simulink subsystem "Charger"  (R2023a)
settings: Solver=VariableStepAuto  StartTime=0.0  StopTime=10.0  RelTol=1e-3
undefined symbols (not defined in the file): SRE, ts
libraries: fl_lib x2, simulink x1, nesl_utility_internal x1
settings Model: Creator=The MathWorks, Inc.  LastModifiedBy=The MathWorks, Inc.
settings SolverCC: AlgebraicLoopSolver=TrustRegion  MaxZcPerStep=1
settings OptimizationCC: ReuseModelBlockBuffer=off
settings DebuggingCC: UnconnectedInputMsg=warning  UnconnectedOutputMsg=warning  UnconnectedLineMsg=warning
settings ModelReferenceCC: EnableRefExpFcnMdlSchedulingChecks=on
settings RTWCC: DLArmComputeVersion=19.05

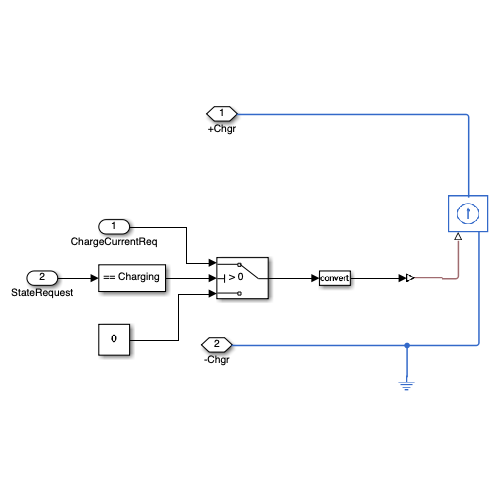
[thumbnail: Simulink's stored preview of the top-level diagram]
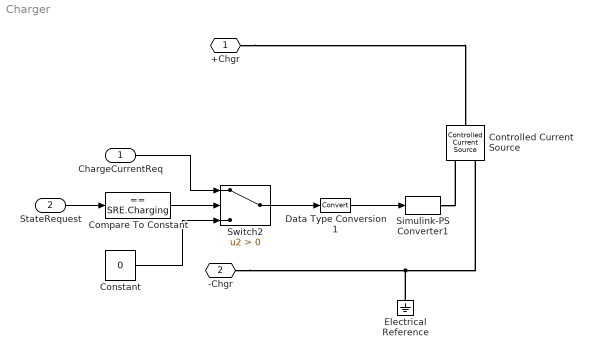
== system Charger ==
  ChargeCurrentReq : Inport
  StateRequest : Inport  Port=2
  Compare To Constant : simulink/Logic and Bit Operations/Compare To Constant  relop===  const=SRE.Charging  OutDataTypeStr=boolean
  Constant : Constant  Value=0  SampleTime=ts
  Controlled Current Source : fl_lib/Electrical/Electrical Sources/Controlled Current Source
      settings: SourceProductName=Foundation Library  LogSimulationData=on
  Data Type Conversion1 : DataTypeConversion  SaturateOnIntegerOverflow=off  RndMeth=Floor
  Electrical Reference : fl_lib/Electrical/Electrical Elements/Electrical Reference
      settings: SourceProductName=Foundation Library
  Simulink-PS Converter1 : nesl_utility_internal/Simulink-PS Converter  PhysicalDomain=network_engine_domain  SubClassName=ps_input  LeftPortType=input  RightPortType=output  PseudoPeriodic=off  Frequencies=[]  NoiseDistribution=none  NoiseParameters=[]  Unit=1  AffineConversion=off  FilteringAndDerivatives=zero  SimscapeFilterOrder=1  InputFilterTimeConstant=0.001  UdotUserProvided=1
  Switch2 : Switch  Criteria=u2 > Threshold  SaturateOnIntegerOverflow=off  InputSameDT=off
  +Chgr : PMIOPort  Side=Left
  -Chgr : PMIOPort  Port=2  Side=Left
  wires:
  Switch2/1 -> Data Type Conversion1/1
  StateRequest/1 -> Compare To Constant/1
  ChargeCurrentReq/1 -> Switch2/1
  Compare To Constant/1 -> Switch2/2
  Data Type Conversion1/1 -> Simulink-PS Converter1/1
  Constant/1 -> Switch2/3
  connections:
  Controlled Current Source/RConn2 -- -Chgr/RConn1 -- Electrical Reference/LConn1
  +Chgr/RConn1 -- Controlled Current Source/LConn1
  Simulink-PS Converter1/RConn1 -- Controlled Current Source/RConn1
